simulink library "Pipe_Geometry"  (Simulink 8.2)
settings: Solver=ode45  StartTime=0.0  StopTime=10.0  RelTol=1e-3
libraries: carnot x4
settings Model: Creator=lena.frank  LastModifiedBy=drhf

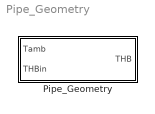
== system Pipe_Geometry ==
  Pipe_Geometry : Subsystem  mask(Pipe Geometry){dia=0.02, len=10, hgt=10, uloss=100/20/10, cond=0, cwall=1000, t0=20, rough=0.04*1e-3, nbend=4, nodes=1}
      mask prompts: dia "diameter [m]"; len "length of pipe [m]"; hgt "static height [m], (positive for outlet above inlet)"; uloss "heat loss per length of pipe [W/(m*K)]"; cond "effective conductivity in the pipe [W/(m*K)]"; cwall "capacity of pipewall per length [J/(m*K)]"; t0 "initial temperature [degree centigrade]"; rough "roughness of pipe [m]"; nbend "number of 90° bends (45° = 0.667)"; nodes "number of nodes"
      mask help:
      | Multinode pipe with capacity and theoretical pressure drop calculation. The flow is calculated by the upwind scheme heat conduction between nodes by central differences (Patankar 1980).
      | heat loss: ul = 2*Conductivity*pi*d_in*Length/Length/(d_in*ln(d_out/d_in))
      | The pressure change due to static height can usually be neglected for closes loop pumped systems.
      mask init:
      | if dia < 0.001
      |     dia = 0.001;
      |     disp('Warning in Pipe: diameter set to minimum value 0.001 m')
      | end
      | if len < 0.001
      |     len = 0.001;
      |     disp('Warning in Pipe: length set to minimum value 0.001 m')
      | end
      | if cwall < 0.001
      |     cwall = 0.001;
      |     disp('Warning in Pipe: heat capacity of the wall set to minimum value 0.001 m')
      | end
      | if nodes < 1
      |     nodes = 1;
      |     disp('Warning in Pipe: number of nodes set to minimum 1')
      | end
      | if nbend < 0
      |     nbend = 0;
      |     disp('Warning in Pipe: number of bends set to minimum 0')
      | end
      | if rough < 0
      |     rough = 0;
      |     disp('Warning in Pipe: roughness of nodes set to minimum 0 m')
      | end
      mask Help: web(fullfile(path_carnot('help'),'Pipe_Geometry.html'),'-helpbrowser')
      mask Display: plot(0,0,90,100,[8,12,16,16,12,8,8],[46,38,46,55,62,55,46],[12,33,48,52,70,73,73,70,50,35,30,12],[38,49,30,30,50,55,65,70,50,70,70,62])

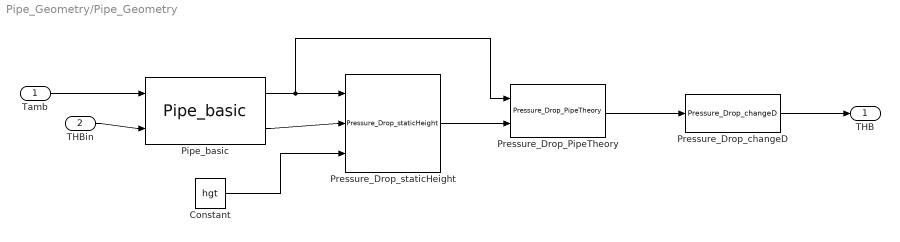
== system Pipe_Geometry/Pipe_Geometry ==
  Tamb : Inport
  THBin : Inport  Port=2
  Constant : Constant  Value=hgt
  Pipe_basic : carnot/Basic/Thermal_Models/Pipe_basic  vol=pi*(dia/2)^2*len  L=len  uloss=uloss  effcond=cond  cwall=cwall  t0=t0  nodes=nodes
  Pressure_Drop_PipeTheory : carnot/Basic/Pressure_Drop/Pressure_Drop_PipeTheory  dia=dia  len=len  rough=rough  nbend=nbend
  Pressure_Drop_changeD : carnot/Basic/Pressure_Drop/Pressure_Drop_changeD  dia=dia
  Pressure_Drop_staticHeight : carnot/Basic/Pressure_Drop/Pressure_Drop_staticHeight
  THB : Outport
  wires:
  Tamb/1 -> Pipe_basic/1
  THBin/1 -> Pipe_basic/2
  Pipe_basic/1 -> Pressure_Drop_staticHeight/1, Pressure_Drop_PipeTheory/1
  Pipe_basic/2 -> Pressure_Drop_staticHeight/2
  Constant/1 -> Pressure_Drop_staticHeight/3
  Pressure_Drop_changeD/1 -> THB/1
  Pressure_Drop_staticHeight/1 -> Pressure_Drop_PipeTheory/2
  Pressure_Drop_PipeTheory/1 -> Pressure_Drop_changeD/1
